simulink model "Test_Ralenti_BO_End_New"  (Simulink 6.5)
settings: Solver=ode45  SolverMode=SingleTasking  StartTime=0.0  StopTime=80  FixedStep=10e-3  MaxStep=0.01  RelTol=1e-5  AbsTol=1e-6
undefined symbols (not defined in the file): AaNeTest, NeTest, NeTimeTest, PcolNeTest, SectionBpNeTest, x
settings Model: Creator=a030141  LastModifiedBy=Zeus
settings DataIOCC: LimitDataPoints=off  SignalLoggingName=sigsOut
settings OptimizationCC: BlockReduction=off  BooleanDataType=off
settings DebuggingCC: SolverPrmCheckMsg=none  MultiTaskDSMMsg=warning  MultiTaskCondExecSysMsg=none  StrictBusMsg=None
settings HardwareCC: TargetUnknown=on
settings RTWCC: TemplateMakefile=grt_vc.tmf  IncludeERTFirstTime=on

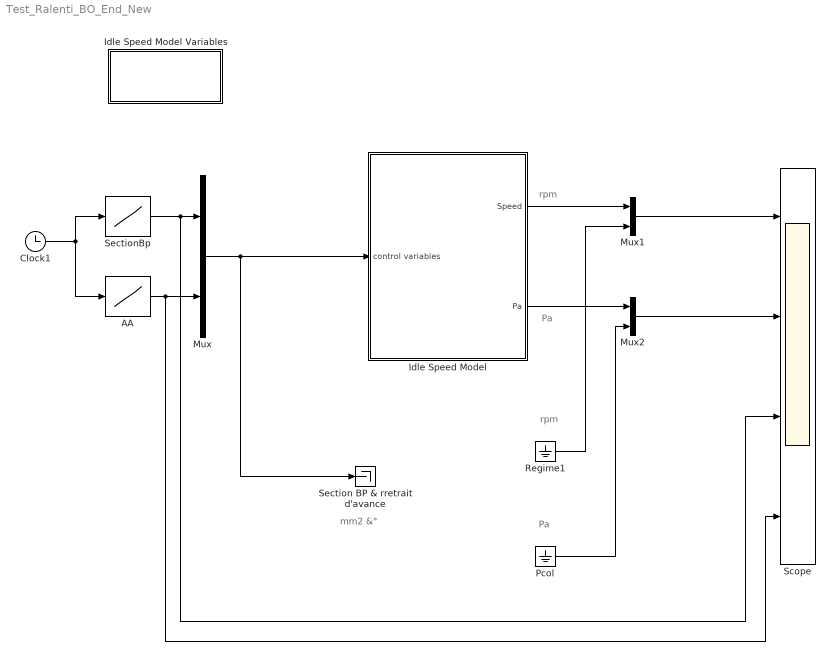
== system Test_Ralenti_BO_End_New ==
  note: Pa
  note: rpm
  note: mm2 &°
  note: rpm
  note: Pa
  AA : Lookup  InputValues=NeTimeTest  OutputValues=AaNeTest  LookUpMeth=Interpolation-Extrapolation  OutDataType=sfix(16)  OutScaling=2^0  SaturateOnIntegerOverflow=on  SampleTime=-1  LUTDesignTableMode=Redesign Table  LUTDesignDataSource=Block Dialog  LUTDesignFunctionName=sqrt(x)  LUTDesignUseExistingBP=on  LUTDesignRelError=0.01  LUTDesignAbsError=1e-6  RndMeth=Floor
      settings: LockScale=off
  Clock1 : Clock
      settings: Decimation=10
  Idle Speed Model : Subsystem
      mask Display: disp('ENGINE MODEL\nLF -> event stroke')
  Idle Speed Model Variables : Subsystem
      mask Display: disp('Load\nDisturbances')
  Mux : Mux  Inputs=2
  Mux1 : Mux  Inputs=2
  Mux2 : Mux  Inputs=2
  Pcol : Ground
  Regime1 : Ground
  Scope : Scope  NumInputPorts=4
      settings: YMin=-5~-5~-5~-5  YMax=5~5~5~5
  Section BP & rretrait d'avance : Terminator
  SectionBp : Lookup  InputValues=NeTimeTest  OutputValues=SectionBpNeTest  LookUpMeth=Interpolation-Extrapolation  OutDataType=sfix(16)  OutScaling=2^0  SaturateOnIntegerOverflow=on  SampleTime=-1  LUTDesignTableMode=Redesign Table  LUTDesignDataSource=Block Dialog  LUTDesignFunctionName=sqrt(x)  LUTDesignUseExistingBP=on  LUTDesignRelError=0.01  LUTDesignAbsError=1e-6  RndMeth=Floor
      settings: LockScale=off
  wires:
  Mux/1 -> Idle Speed Model/1(control variables), Section BP & rretrait d'avance/1
  SectionBp/1 -> Mux/1, Scope/3
  AA/1 -> Mux/2, Scope/4
  Clock1/1 -> SectionBp/1, AA/1
  Idle Speed Model/1(Speed) -> Mux1/1
  Mux1/1 -> Scope/1
  Idle Speed Model/2(Pa) -> Mux2/1
  Mux2/1 -> Scope/2
  Regime1/1 -> Mux1/2
  Pcol/1 -> Mux2/2

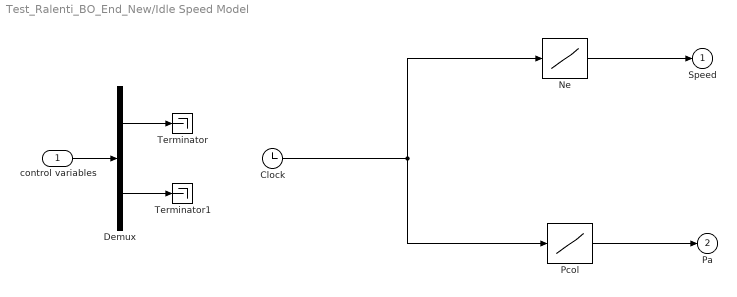
== system Test_Ralenti_BO_End_New/Idle Speed Model ==
  control variables : Inport
  Clock : Clock
      settings: Decimation=10
  Demux : Demux  Outputs=2
  Ne : Lookup  InputValues=NeTimeTest  OutputValues=NeTest  LookUpMeth=Interpolation-Extrapolation  OutDataType=sfix(16)  OutScaling=2^0  SaturateOnIntegerOverflow=on  SampleTime=-1  LUTDesignTableMode=Redesign Table  LUTDesignDataSource=Block Dialog  LUTDesignFunctionName=sqrt(x)  LUTDesignUseExistingBP=on  LUTDesignRelError=0.01  LUTDesignAbsError=1e-6  RndMeth=Floor
      settings: LockScale=off
  Pcol : Lookup  InputValues=NeTimeTest  OutputValues=PcolNeTest  LookUpMeth=Interpolation-Extrapolation  OutDataType=sfix(16)  OutScaling=2^0  SaturateOnIntegerOverflow=on  SampleTime=-1  LUTDesignTableMode=Redesign Table  LUTDesignDataSource=Block Dialog  LUTDesignFunctionName=sqrt(x)  LUTDesignUseExistingBP=on  LUTDesignRelError=0.01  LUTDesignAbsError=1e-6  RndMeth=Floor
      settings: LockScale=off
  Terminator : Terminator
  Terminator1 : Terminator
  Speed : Outport
  Pa : Outport  Port=2
  wires:
  Demux/1 -> Terminator/1
  control variables/1 -> Demux/1
  Ne/1 -> Speed/1
  Pcol/1 -> Pa/1
  Clock/1 -> Ne/1, Pcol/1
  Demux/2 -> Terminator1/1

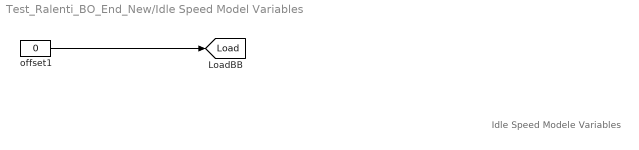
== system Test_Ralenti_BO_End_New/Idle Speed Model Variables ==
  note: Idle Speed Modele Variables
  offset1 : Constant  Value=0  OutDataType=sfix(16)  ConRadixGroup=Use specified scaling  OutScaling=2^0  SampleTime=inf  FramePeriod=inf
  tag scope: Load=global
  wires:
  offset1/1 -> [Load]
